simulink model "template_linear"  (Simulink 7.2)
settings: Solver=ode1  StartTime=0.0  StopTime=inf  FixedStep=0.002  RelTol=1e-3
PostLoadFcn:
  | qc_set_target_type(getConfigSet(bdroot, 'QUARC Default Target Configuration'));
undefined symbols (not defined in the file or in its folder): HIL
libraries: quarc_library x3, simulink x1
settings Model: Creator=pmartin  LastModifiedBy=controle  SimulationMode=external  ExtModeTrigDuration=5000
settings SolverCC: PositivePriorityOrder=on
settings OptimizationCC: InitFltsAndDblsToZero=on
settings DebuggingCC: SaveWithParameterizedLinksMsg=none  MultiTaskDSMMsg=warning  MultiTaskCondExecSysMsg=none  StrictBusMsg=None
settings RTWCC: SystemTargetFile=quarc_windows.tlc  TemplateMakefile=quarc_default_tmf  Description=QUARC Win32 Target  ProcessScript=quarc_windows_make_rtw_hook
settings STFCustomTargetCC: TargetPreCompLibLocation=C:\DOCUME~1\ALLUSE~1\DADOSD~1\QUARC\lib\2008b\windows\release  SystemTargetFile=quarc_windows.tlc
settings GRTTargetCC: TargetPreCompLibLocation=C:\DOCUME~1\ALLUSE~1\DADOSD~1\QUARC\lib\2008b\windows\release  CompOptLevelCompliant=off  MatFileLogging=off  ExtMode=on  ExtModeMexFile=quarc_comm

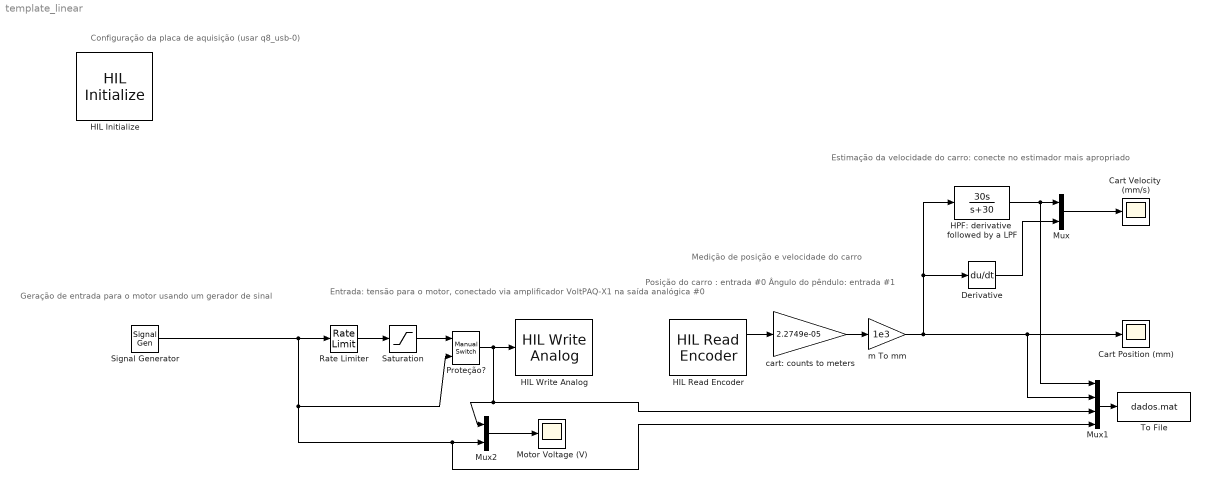
== system template_linear ==
  note: Posição do carro : entrada #0
      | Ângulo do pêndulo: entrada #1
  note: Estimação da velocidade do carro:
      | conecte no estimador mais apropriado
  note: Entrada: tensão para o motor, conectado via
      | amplificador VoltPAQ-X1 na saída analógica #0
  note: Configuração da placa de aquisição (usar q8_usb-0)
  note: Medição de posição e velocidade do carro
  note: Geração de entrada para o motor
      | usando um gerador de sinal
  Cart Position (mm) : Scope
      settings: TickLabels=on  TimeRange=10  YMin=10  YMax=180  SaveName=data_xc  DataFormat=Array
  Cart Velocity  (mm/s) : Scope
      settings: TickLabels=on  TimeRange=10  YMin=-350  YMax=350  SaveName=data_xc1  DataFormat=Array
  Derivative : Derivative
  HIL Initialize : quarc_library/Data Acquisition/Generic/Configuration/HIL Initialize  object_name=HIL-1  board_type=q8_usb  board_number=0  board_options=update_rate=normal  exclusive=off  active=off  hardware_clocks=[0:2]  clock_modes=[]  set_clock_params_at_start=off  set_clock_params_at_switch_in=off  analog_input_channels=[0:7]  analog_input_maximums=10  analog_input_minimums=-10  set_analog_input_params_at_start=on  set_analog_input_params_at_switch_in=off  analog_output_channels=[0:7]  analog_output_maximums=10  analog_output_minimums=-10  initial_analog_outputs=[0]  final_analog_outputs=[0]  watchdog_analog_outputs=0  set_analog_output_params_at_start=on  set_analog_output_params_at_switch_in=off  set_analog_outputs_at_start=on  set_analog_outputs_at_switch_in=off  set_analog_outputs_at_terminate=on  set_analog_outputs_at_switch_out=off  set_analog_outputs_on_watchdog=off  digital_input_channels=[]  digital_output_channels=[0:7]  digital_output_configuration=[]  initial_digital_outputs=[0]  final_digital_outputs=[0]  watchdog_digital_outputs=[0]  set_digital_output_params_at_start=off  set_digital_output_params_at_switch_in=off  set_digital_outputs_at_start=on  set_digital_outputs_at_switch_in=off  set_digital_outputs_at_terminate=on  set_digital_outputs_at_switch_out=off  set_digital_outputs_on_watchdog=off  encoder_channels=[0:7]  quadrature=[4]  encoder_filter_frequency=[]  initial_encoder_counts=[0]  set_encoder_params_at_start=on  set_encoder_params_at_switch_in=off  set_encoder_counts_at_start=on  set_encoder_counts_at_switch_in=off  pwm_channels=[0:7]  pwm_modes=0  pwm_frequency=99.532799999999995e6/4095  pwm_configuration=[0]  pwm_alignment=[0]  pwm_polarity=[1]  pwm_leading_deadband=[0]  pwm_trailing_deadband=[0]  initial_pwm_outputs=[0]  final_pwm_outputs=[0]  watchdog_pwm_outputs=[0]  set_pwm_params_at_start=on  set_pwm_params_at_switch_in=off  set_pwm_outputs_at_start=on  set_pwm_outputs_at_switch_in=off  set_pwm_outputs_at_terminate=on  set_pwm_outputs_at_switch_out=off  set_pwm_outputs_on_watchdog=off  other_output_channels=[]  initial_other_outputs=[]  final_other_outputs=[]  watchdog_other_outputs=[]  set_other_outputs_at_start=off  set_other_outputs_at_switch_in=off  set_other_outputs_at_terminate=off  set_other_outputs_at_switch_out=off  set_other_outputs_on_watchdog=off
  HIL Read Encoder : quarc_library/Data Acquisition/Generic/Immediate I//O/HIL Read Encoder  object_name=HIL-1  channels=[0:1]  sample_time=qc_get_step_size  active=on  vector_output=off  data_type_mode=Inherit via back propagation  data_type=double
  HIL Write Analog : quarc_library/Data Acquisition/Generic/Immediate I//O/HIL Write Analog  object_name=HIL-1  channels=0  sample_time=-1  active=off  vector_input=off
  HPF: derivative  followed by a LPF : TransferFcn  Numerator=[30 0]  Denominator=[1 30]
  Motor Voltage (V) : Scope
  Mux : Mux  Inputs=2
  Mux1 : Mux
  Mux2 : Mux  Inputs=2
  Proteção? : simulink/Signal Routing/Manual Switch  SystemSampleTime=-1  sw=1  action=0  varsize=off
  Rate Limiter : RateLimiter  RisingSlewLimit=40  FallingSlewLimit=-40  SampleTimeMode=inherited
  Saturation : Saturate  UpperLimit=7.2  LowerLimit=-7.2  OutDataType=sfix(16)  OutScaling=2^0
  Signal Generator : SignalGenerator  WaveForm=square  Amplitude=2  Frequency=0.5
  To File : ToFile  Filename=dados.mat  MatrixName=dados
  cart: counts to meters : Gain  Gain=2.2749e-05  SaturateOnIntegerOverflow=on  OutDataTypeStr=Inherit: Same as input  ParamDataTypeStr=Inherit: Same as input
  m To mm : Gain  Gain=1e3  SaturateOnIntegerOverflow=on  OutDataTypeStr=Inherit: Same as input  ParamDataTypeStr=Inherit: Same as input
  wires:
  m To mm/1 -> Derivative/1, HPF: derivative  followed by a LPF/1, Cart Position (mm)/1, Mux1/2
  HIL Read Encoder/1 -> cart: counts to meters/1
  cart: counts to meters/1 -> m To mm/1
  HPF: derivative  followed by a LPF/1 -> Mux/1, Mux1/1
  Derivative/1 -> Mux/2
  Mux/1 -> Cart Velocity  (mm/s)/1
  Mux1/1 -> To File/1
  Saturation/1 -> Proteção?/1
  Proteção?/1 -> HIL Write Analog/1, Mux2/1, Mux1/3
  Rate Limiter/1 -> Saturation/1
  Signal Generator/1 -> Rate Limiter/1, Proteção?/2, Mux2/2, Mux1/4
  Mux2/1 -> Motor Voltage (V)/1
